simulink model "CameraExample"  (R2014b)
settings: Solver=FixedStepDiscrete  StartTime=0.0  StopTime=inf  RelTol=1e-3
settings Model: Creator=aurora  LastModifiedBy=aurora
settings DataIOCC: LimitDataPoints=off  SaveOutput=off  SaveTime=off
settings OptimizationCC: SimCompilerOptimization=On

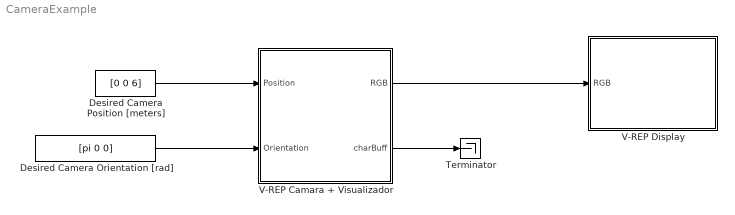
== system CameraExample ==
  Desired Camera Orientation [rad] : Constant  Value=[pi 0 0]  OutDataTypeStr=single
  Desired Camera Position [meters] : Constant  Value=[0 0 6]  OutDataTypeStr=single
  Terminator : Terminator
  V-REP Camara + Visualizador : Subsystem  mask{ResX=512, ResY=512, id=4}
      mask prompts: ResX "Camera  X resolution"; ResY "Camera Y resolution"; id "Share Memory Id"
      mask Display:
      | image('webcam.jpg')
      | color('red');
      | port_label('input',1,'Position')
      | port_label('input',2,'Orientation')
      | port_label('output',1,'RGB')
      | port_label('output',2,'Char Buffer')
  V-REP Display : Subsystem  mask{ResX=512, ResY=512, id=11}
      mask prompts: ResX "Display X resolution"; ResY "Display Y resolution"; id "Share Memory Id"
      mask Display:
      | image('display.jpg')
      | color('white');
      | port_label('input',1,'RGB')
  wires:
  V-REP Camara + Visualizador/1(RGB) -> V-REP Display/1("RGB ")
  Desired Camera Position [meters]/1 -> V-REP Camara + Visualizador/1("Position ")
  Desired Camera Orientation [rad]/1 -> V-REP Camara + Visualizador/2(Orientation)
  V-REP Camara + Visualizador/2(charBuff) -> Terminator/1

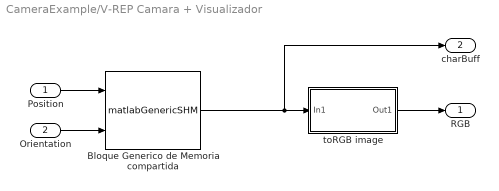
== system CameraExample/V-REP Camara + Visualizador ==
  "Position " : Inport
  Orientation : Inport  Port=2
  Bloque Generico de Memoria compartida : S-Function  FunctionName=matlabGenericSHM  Parameters=nombre,dispositivo,vecE,vecS,tipoE,tipoS  EnableBusSupport=off  mask(Bloque Generico Memoria Compartida V1.1){nombre='vrepCam', dispositivo=id, vecE=[3 3], vecS=[3*ResX*ResY], tipoE=['f' 'f'], tipoS=['C']}
      mask prompts: nombre "Nombre Base de la Memoria"; dispositivo "Numero de Dispositivo"; vecE "Vector de Entradas"; vecS "Vector de Salidas"; tipoE "Tipo de dato Entradas"; tipoS "Tipo de datos Salidas"
      mask help:
      | Este bloque permite la creacion simultanea de una memoria compartida de entrada y una memoria compartida de Salida con una estructura definida por el usuario.
      | Es compatible en Windows y Linux. Para mas informacion ver ayuda.
      mask Help:
      | Nombre Base de Memoria (nombre): Es el string base de la memoria compartida ej 'robot'
      | Numero de Dispositivo (dispositivo): entero que identifica el dispositivo entre varios en uso
      | Se crean dos memorias compartidas con el nombre:
      | "%name_entrada_%dispositivo" para la entrada al dispositivo (escritura)
      | "%name_salida_%dispositivo" para la salida del dispositivo (lectura)
      | Vector de Entradas (vecE): arreglo que especifica la cantidad de entradas y su dimension
      | Vector de Salidas  (vecS): arreglo que especifica la cantidad de entradas y su dimension
      | Tipo Entradas(tipoE): arreglo de caracteres que indica el tipo de cada entrada
      | Tipo Salidas (tipoS): arreglo de caracteres que indica el tipo de cada salida
      | Los tipos pueden ser de la siguiente forma:
      | ('f'=float, 'd'=double, 'i'=int32, 'c'=char, 'C'= unsigned char, 'I'=unsigned int)
      | Ejemplo.
      | Suponer los siguientes parametros:
      | nombre='memoriaEjemplo'
      | dispositivo=10
      | vecE=[3 2 1]
      | vecS=[6 5 7 8]
      | tipoE=['f' 'I' 'c']
      | tipoS=['C' 'i' 'd' 'd']
      | 
      | Crean dos memorias compartidas denominadas :
      | "%memoriaEjemplo_entrada_10" (entrada al bloque)
      | "%memoriaEjemplo_salida_10"  (salida del bloque)
      | Se crean 3 entradas:
      |  1° Dimension 3 y tipo "unsigned char"
      |  2° Dimension 2 y tipo "int"
      |  3° Dimension 1 y tipo "char"
      | Se crean 4 salidas:
      |  1° Dimension 6 y tipo "float"
      |  2° Dimension 5 y tipo "unsigned int"
      |  3° Dimension 7 y tipo "double"
      |  3° Dimension 8 y tipo "double"
      mask Display: image('shareMem.gif')
  toRGB image : Subsystem  mask{ResX=ResX, ResY=ResY}
      mask prompts: ResX "Resolucion Camara X"; ResY "Resolucion Camara Y"
      mask Display:
      | port_label('output', 1, 'RGB')
      | port_label('input', 1, 'videoIN')
  RGB : Outport
  charBuff : Outport  Port=2
  wires:
  Bloque Generico de Memoria compartida/1 -> charBuff/1, toRGB image/1(In1)
  Orientation/1 -> Bloque Generico de Memoria compartida/2
  toRGB image/1(Out1) -> RGB/1
  "Position "/1 -> Bloque Generico de Memoria compartida/1

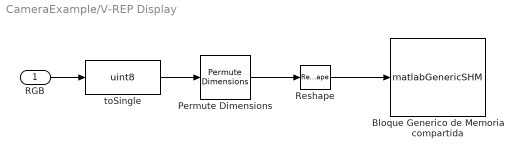
== system CameraExample/V-REP Display ==
  "RGB " : Inport
  Bloque Generico de Memoria compartida : S-Function  FunctionName=matlabGenericSHM  Parameters=nombre,dispositivo,vecE,vecS,tipoE,tipoS  EnableBusSupport=off  mask(Bloque Generico Memoria Compartida V1.1){nombre='vrepDisplay', dispositivo=id, vecE=[3*ResX*ResY], vecS=[], tipoE=['C'], tipoS=[]}
      mask prompts: nombre "Nombre Base de la Memoria"; dispositivo "Numero de Dispositivo"; vecE "Vector de Entradas"; vecS "Vector de Salidas"; tipoE "Tipo de dato Entradas"; tipoS "Tipo de datos Salidas"
      mask help:
      | Este bloque permite la creacion simultanea de una memoria compartida de entrada y una memoria compartida de Salida con una estructura definida por el usuario.
      | Es compatible en Windows y Linux. Para mas informacion ver ayuda.
      mask Help:
      | Nombre Base de Memoria (nombre): Es el string base de la memoria compartida ej 'robot'
      | Numero de Dispositivo (dispositivo): entero que identifica el dispositivo entre varios en uso
      | Se crean dos memorias compartidas con el nombre:
      | "%name_entrada_%dispositivo" para la entrada al dispositivo (escritura)
      | "%name_salida_%dispositivo" para la salida del dispositivo (lectura)
      | Vector de Entradas (vecE): arreglo que especifica la cantidad de entradas y su dimension
      | Vector de Salidas  (vecS): arreglo que especifica la cantidad de entradas y su dimension
      | Tipo Entradas(tipoE): arreglo de caracteres que indica el tipo de cada entrada
      | Tipo Salidas (tipoS): arreglo de caracteres que indica el tipo de cada salida
      | Los tipos pueden ser de la siguiente forma:
      | ('f'=float, 'd'=double, 'i'=int32, 'c'=char, 'C'= unsigned char, 'I'=unsigned int)
      | Ejemplo.
      | Suponer los siguientes parametros:
      | nombre='memoriaEjemplo'
      | dispositivo=10
      | vecE=[3 2 1]
      | vecS=[6 5 7 8]
      | tipoE=['f' 'I' 'c']
      | tipoS=['C' 'i' 'd' 'd']
      | 
      | Crean dos memorias compartidas denominadas :
      | "%memoriaEjemplo_entrada_10" (entrada al bloque)
      | "%memoriaEjemplo_salida_10"  (salida del bloque)
      | Se crean 3 entradas:
      |  1° Dimension 3 y tipo "unsigned char"
      |  2° Dimension 2 y tipo "int"
      |  3° Dimension 1 y tipo "char"
      | Se crean 4 salidas:
      |  1° Dimension 6 y tipo "float"
      |  2° Dimension 5 y tipo "unsigned int"
      |  3° Dimension 7 y tipo "double"
      |  3° Dimension 8 y tipo "double"
      mask Display: image('shareMem.gif')
  Permute Dimensions : PermuteDimensions  Order=[3,2,1]
  Reshape : Reshape
  toSingle : DataTypeConversion  OutDataTypeStr=uint8
  wires:
  toSingle/1 -> Permute Dimensions/1
  "RGB "/1 -> toSingle/1
  Reshape/1 -> Bloque Generico de Memoria compartida/1
  Permute Dimensions/1 -> Reshape/1

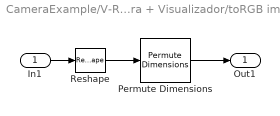
== system CameraExample/V-REP Camara + Visualizador/toRGB image ==
  In1 : Inport
  Permute Dimensions : PermuteDimensions  Order=[3 2 1]
  Reshape : Reshape  OutputDimensionality=Customize  OutputDimensions=[3,ResX,ResY]
  Out1 : Outport
  wires:
  Permute Dimensions/1 -> Out1/1
  Reshape/1 -> Permute Dimensions/1
  In1/1 -> Reshape/1
